simulink model "s32k344_mcb_open_loop_s32ct"  (R2024b)
settings: Solver=FixedStepAuto  StartTime=0.0  StopTime=10.0  RelTol=1e-3  EnableMultiTasking=on
PreLoadFcn:
  | % NXP_MBDT_S32K3 callback: DO NOT REMOVE
  | mbd_s32k3.common.nxp.model_callbacks.preLoadFcn();
  | 
  | s32k344Data;
  | mcbOpenLoopData;
PostLoadFcn:
  | % NXP_MBDT_S32K3 callback: DO NOT REMOVE
  | mbd_s32k3.common.nxp.model_callbacks.postLoadFcn();
InitFcn:
  | % NXP_MBDT_S32K3 callback: DO NOT REMOVE
  | mbd_s32k3.common.nxp.model_callbacks.initFcn();
values from neighbouring files (symbols this model uses):
  PWM_DutyScale = 32768    [s32k344Data.m]
  PWM_Period = 8000    [s32k344Data.m]
  Ts_motor = T_pwm    (= 5e-05)    [s32k344Data.m]
undefined symbols (not defined in the file or in its folder): inverter, LogicOutputId, pmsm, Value
libraries: mbd_s32k3_io_library x14, mbd_s32k3_cdd_library x4, simulink x4, mbd_s32k3_isr_library x1, mbd_s32k3_utility_library x1
(part 1 of 3)
Description:
  | Motor Control PMSM Open Loop MCB S32CT
  | 
  | 
  |             <script src="../../../../doc/src/utils.js">
  | 
  |             <script src="../../../../doc/src/details_summary_utils.js">
  | 
  |             <script src="../../../../doc/src/matlab_command_link.js">
  | 
  |             <link rel="stylesheet" type="text/css" href="../../../../doc/style.css">
  | 
  | 
  | 
  | 
  |         Motor Control PMSM Open Loop MCB S32CT
  |         <a class="matlab-command" href="matlab:open('s32k344_mcb_open_loop_s32ct')"><button class="matlab-command" style=" --data-title: ' Run MATLAB command: open(\'s32k344_mcb_open_loop_s32ct')'">Open Example
  |         The s32k344_mcb_open_loop_s32ct.mdl example illustrates how the MCSPTE1AK344 Motor Control Development Kit is used to run a motor by achieving an open-loop control algorithm (also known as scalar control or V/Hz control). This technique varies the stator voltage and frequency to control the rotor speed without using any feedback from the motor. Open-Loop control does not have the ability to consider the external conditions that can affect the motor speed. Therefore, the control system cannot automatically correct the deviation between the desired and the actual motor speed. This Simulink® model is configured to work with both Sunrise 42BLY3A78-24110 and Linix 45ZWN24-40 motors and it has been tested on the S32K3X4EVB-Q172 RevA board.
  | 
  |             This model shows how to get started with Motor Control Blockset™ and verify the hardware setup for the MCSPTE1AK344 Development Kit by running the motor. The model algorithm also reads the ADC values for the 3-phase currents and DC Bus voltage, using the hardware triggering scheme of eMIOS-TRGMUX-BCTU-ADC. To generate the output commands for spinning the motor, this model uses the Motor Control Blockset™ Library. The FreeMASTER application is used to connect to the running on-target algorithm using the FreMASTER CMSIS-DAP Communication Plug-in.
  | 
  |             Note: If there is no error, the <b style="color:blue">RGBLED0_BLUE will be on which means the application is waiting for the user commands. If there is any error, the motor will not run, and the <b style="color:red">RGBLED0_RED will stay on. If the motor is spinning and no fault is detected, the <b style="color:green">RGBLED0_GREEN will stay on.
  | 
  |             Note: Make sure to have included in MATLAB Path the mcat_src_files directory!
  | 
  |         Toolchain Supported
  | 
  | 
  |                 S32 Design Studio 3.5
  | 
  | 
  |         Required Hardware
  | 
  | 
  |                 Personal Computer
  | 
  |                 <a href="https://www.nxp.com/design/development-boards/automotive-motor-control-solutions/arm-based-solutions-/s32k344-brushless-direct-current-and-permanent-magnet-synchronous-motor-control-development-kit:MCSPTE1AK344"> MCSPTE1AK344 BLDC and PMSM Motor Control Development Kit<img src="../img/MCSPTE1AK344.jpg" alt="Motor Control PMSM Open Loop MCB S32CT" height="auto"> The MCSPTE1AK344 Development kit contains:  <a href="https://www.nxp.com/design/development-boards/automotive-development-platforms/hardware-tools-accessories/motor-control-shield-for-devkit:DEVKIT-MOTORGD"> DEVKIT-MOTORGD board<a href="https://www.nxp.com/design/design-center/development-boards/automotive-development-platforms/s32k-mcu-platforms/s32k3x4evb-t172-evaluation-board-for-automotive-general-purpose:S32K3X4EVB-T172">S32K3X4EVB-T172 board or <a href="https://www.nxp.com/design/development-boards/automotive-development-platforms/s32k-mcu-platforms/s32k3x4-q172-general-purpose-development-board:S32K3X4EVB-Q172">S32K3X4EVB-Q172 board<a href="https://www.sunrisemotor-cn.com/Product/142451.html"> Sunrise 42BLY3A78-24110 Motor
  | 
  |                 12V Power Supply
  | 
  |                 Micro USB cable
  | 
  | 
  |         Prepare the Demo
  | 
  | 
  |                 The MCSPTE1AK344 kit has different resistors removed/populated compared with the original S32K3X4EVB board. The following table presents all the modifications needed for the S32K3X4EVB boards to work with all MBDT BLDC/PMSM models:<table class="tg" style="undefined;table-layout: fixed; width: 700px"><col style="width: 182.px"><col style="width: 144.px"><col style="width: 112.px"><col style="width: 144.px"><col style="width: 112.px">Board RevisionsRemoved resistorsValue/PackagePopulated resistorsValue/Package<td rowspan="2">S32K3X4EVB-T172R37, R4010k Ohm/0402<td rowspan="2">R255, R257, R2273<td rowspan="2">0 Ohm/0402R22390 Ohm/0402<td rowspan="2">S32K3X4EVB-Q172 RevAR37, R4010k Ohm/0402<td rowspan="2">R255, R257<td rowspan="2">0 Ohm/0402R91, R960 Ohm/0402<td rowspan="2">S32K3X4EVB-Q172 RevBR37, R4010k Ohm/0402<td rowspan="2">R255, R257, R2188<td rowspan="2">0 Ohm/0402R91, R96, R21860 Ohm/0402
  | 
  |                 For more details check the <a href="https://www.nxp.com/webapp/Download?colCode=S32K3X4EVBBMUG&location=null">S32K3X4EVB-Q172 Board Modifications for MCSPTE1AK344 Motor Control Kit Schematic Addendum.
  | 
  |                 To get started on the MCSPTE1AK344 kit visit the website <a href="https://www.nxp.com/document/guide/get-started-with-the-mcspte1ak344-development-kit:GS-MCSPTE1AK344"> Get Started with the MCSPTE1AK344 Development Kit.
  | 
  |                 The connections between the S32K3X4EVB board and the DEVKIT-MOTORGD can be found in the following table:<img src="../img/Headers_pinout.jpg" alt="Motor Control PMSM Open Loop MCB S32CT" height="500px" >
  | 
  |                 Overview of the location of USER_SW0/SW1, RGBLED0, 12 Vin DC power, USB J40 connector, SW1 for powering ON, board jumpers J8, J9, J10, and J11:<img src="../img/MCSPTE1AK344_top.jpg" alt="Motor Control PMSM Open Loop MCB S32CT" height="500px" >
  | 
  |                 Take a closer look and check the DEVKIT-MOTORGD jumpers J9, J10, and J11 are in positions 2-1 and J8 is open, this configuration works with all MBDT BLDC/PMSM models:<img src="../img/PINS_J9_J11.jpg" alt="Motor Control PMSM Open Loop MCB S32CT" height="300px" >
  | 
  |                 Connect a micro-USB cable between the host PC and the OpenSDA USB port (J40) and switch the SW1 to position 2 on the S32K3X4EVB board.
  | 
  |                 Connect the 12V Power supply to the DEVKIT-MOTORGD board and switch the SW1 from the 2 position to the 1 position on the S32K3X4EVB board: <img src="../img/Plug-Power.jpg" alt="Motor Control PMSM Open Loop MCB S32CT" height="300px">
  | 
  |                 The four LEDs next to SW1 will power on and be solid orange, if they are blinking, move the switch from position 1 to 2 and back to position 1 to start the SBC without the active watchdog.
  | 
  |                 Open the s32k344_mcb_open_loop_s32ct.mdl model.Users can choose between the Sunrise 42BLY3A78-24110 or the Linix 45ZWN24-40 motor from <a href="https://www.nxp.com/design/design-center/development-boards-and-designs/general-purpose-mcus/low-voltage-3-phase-motor-for-frdm-platform:FRDM-MC-LVMTR"> the NXP page.
  | 
  |                 Click on "Generate Code, Build & Deploy" to download the program to the target board and the <b style="color:blue">RGBLED0_BLUE lights up.
  | 
  |                 To open the FreeMASTER software click on "4. Open the FreeMASTER project" from inside the Simulink model, this will open the "s32k344_mcb_open_loop_s32ct.pmpx" file in the "FreeMASTER_control" folder.
  | 
  |                 Click on the "GO" buton (or press CTRL+G) to enable FreeMASTER communication with the S32K3X4EVB board:<img src="../img/FM_Start.jpg" alt="Motor Control PMSM Open Loop MCB S32CT" height="150px"> Successful communication displays in the status bar at the bottom as: RS232; port = COMn; speed = 115200.
  | 
  | 
  |         Running the Demo
  | 
  | 
  |                 To validate this example, please follow the steps below:   To start the motor, set the Enable variable from 0 to 1. The Desired speed can be set from FreeMASTER project with values between -1000 and 1000 RPM The DC Bus voltage, 3-phase currents and generated PWM signals could be also checked in FreeMASTER; The <b style="color:green">RGBLED0_GREEN will be ON when the motor spins:<img src="../img/PMSM.gif" alt="Motor Control PMSM Open Loop MCB S32CT" height="100">
  | 
  | 
  |         Customization Options
  | 
  | 
  |                 For changing the processor, the configuration tool, and for creating custom configuration projects, please visit section 3.6 of Release Notes <a class="pdf-link" href="../../../../doc/docs/manual/Model_Based_Design_Toolbox_S32K3_Series_Release_Notes.pdf">Model_Based_Design_Toolbox_S32K3_Series_Release_Notes.pdf
  | 
  |                 For S32K3 Design Tools and Files, please visit <a href="https://www.nxp.com/products/processors-and-microcontrollers/arm-microcontrollers/s32k-automotive-mcus/s32k3-microcontrollers-for-general-purpose:S32K3">S32K3 Microcontrollers
settings Model: DataDictionary=s32k344_mcb_open_loop_s32ct.sldd  Creator=nxf35401  LastModifiedBy=nxf64875
settings SolverCC: AlgebraicLoopSolver=TrustRegion
settings DataIOCC: LimitDataPoints=on  SaveFormat=Array  SaveOutput=off  SaveTime=off  ReturnWorkspaceOutputs=off
settings OptimizationCC: DefaultParameterBehavior=Inlined  UseFloatMulNetSlope=on  DefaultUnderspecifiedDataType=single  EnhancedBackFolding=on  PassReuseOutputArgsAs=Individual arguments  ZeroExternalMemoryAtStartup=off  ZeroInternalMemoryAtStartup=off  NoFixptDivByZeroProtection=on  EfficientFloat2IntCast=on  MaxStackSize=128  SimCompilerOptimization=on  EfficientTunableParamExpr=on
settings DebuggingCC: InheritedTsInSrcMsg=none  MultiTaskDSMMsg=none  MultiTaskRateTransMsg=warning  ParameterPrecisionLossMsg=none  ParameterTunabilityLossMsg=error  UnconnectedInputMsg=warning  UnconnectedOutputMsg=warning  UnconnectedLineMsg=warning
settings HardwareCC: ProdBitPerPointer=32  ProdBitPerSizeT=32  ProdBitPerPtrDiffT=32  ProdLargestAtomicInteger=Long  ProdLargestAtomicFloat=Double  ProdWordSize=32  ProdHWDeviceType=ARM Compatible->ARM Cortex
settings ModelReferenceCC: EnableRefExpFcnMdlSchedulingChecks=on
settings SFSimCC: MATLABDynamicMemAlloc=off
settings RTWCC: Description=Embedded Coder  SystemTargetFile=ert.tlc  HardwareBoard=NXP S32K3xx  TemplateMakefile=ert_default_tmf  Toolchain=S32DS GCC  BuildConfiguration=Faster Runs  IncludeHyperlinkInReport=on  GPUComputeCapability=3.5  DLArmComputeVersion=19.05
settings CodeAppCC: ForceParamTrailComments=on  IgnoreCustomStorageClasses=off  OperatorAnnotations=on  SimulinkDataObjDesc=on  SFDataObjDesc=on  InsertBlockDesc=on  StateflowObjectComments=on
settings ERTTargetCC: TargetLangStandard=C99 (ISO)  SupportNonFinite=off  SupportComplex=off  InlinedParameterPlacement=Hierarchical  ERTSrcFileBannerTemplate=mbd_s32k3_ert_code_template.cgt  ERTHdrFileBannerTemplate=mbd_s32k3_ert_code_template.cgt  ERTDataSrcFileTemplate=mbd_s32k3_ert_code_template.cgt  ERTDataHdrFileTemplate=mbd_s32k3_ert_code_template.cgt  DynamicArrayContainerType=coder::array

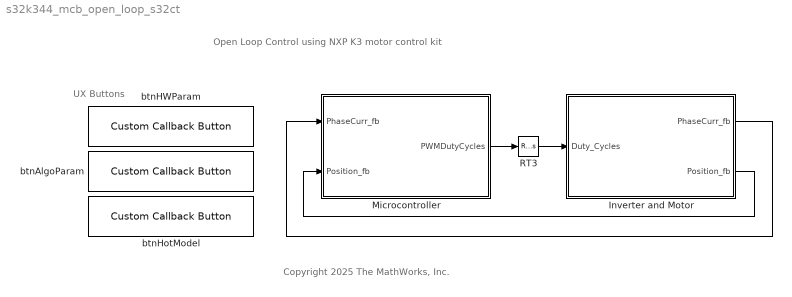
== system s32k344_mcb_open_loop_s32ct ==
  note: UX Buttons
  note: Open Loop Control using NXP K3 motor control kit
  note: Copyright 2025 The MathWorks, Inc.
  Inverter and Motor : Subsystem
  Microcontroller : Subsystem
  RT3 : RateTransition  Integrity=off
  btnAlgoParam : CustomCallbackButton  Configuration="{\"components\":[{\"name\":\"BackgroundImageComponent\",\"settings\":{\"image\":{\"size\":[0,0],\"src\":\"default\",\"srcOrientation\":\"Right\"},\"position\":[0,0,1,1]}},{\"name\":\"ButtonStateComponent\",\"settings\":{\"buttonType\":\"momentary\",\"clickFcn\":\"edit mcbOpenLoopData.m;\",\"onValue\":1,\"position\":[0,0,1,1],\"pressDelay\":\"500\",\"pressFcn\":\"\",\"repeatInterval\":\"0\",\"states\":[{\"horizontalAlignment\":\"center\",\"image\":{\"position\":[0,0,1,1],\"size\":[1,1],\"src\":\"default\",\"srcOrientation\":\"Right\"},\"label\":{\"color\":[0.01176470588,0.01176470588,0.01176470588,1],\"icon\":{\"size\":[0,0],\"src\":\"default\",\"srcOrientation\":\"Right\"},\"iconOffset\":0,\"iconPlacement\":\"left\",\"opacity\":1,\"show\":true,\"text\":{\"content\":\"Edit motor and algorithm parameters\",\"font\":\"Helvetica\"}},\"labelOffset\":[0,0],\"verticalAlignment\":\"middle\"},{\"horizontalAlignment\":\"center\",\"image\":{\"position\":[0,0,1,1],\"size\":[1,1],\"src\":\"default\",\"srcOrientation\":\"Right\"},\"label\":{\"color\":[0.01176470588,0.01176470588,0.01176470588,1],\"icon\":{\"size\":[0,0],\"src\":\"default\",\"srcOrientation\":\"Right\"},\"iconOffset\":0,\"iconPlacement\":\"left\",\"opacity\":1,\"show\":true,\"text\":{\"content\":\"Edit motor and algorithm parameters\",\"font\":\"Helvetica\"}},\"labelOffset\":[0,0],\"verticalAlignment\":\"middle\"},{\"horizontalAlignment\":\"center\",\"image\":{\"position\":[0,0,1,1],\"size\":[1,1],\"src\":\"default\",\"srcOrientation\":\"Right\"},\"label\":{\"color\":[0.01176470588,0.01176470588,0.01176470588,1],\"icon\":{\"size\":[0,0],\"src\":\"default\",\"srcOrientation\":\"Right\"},\"iconOffset\":0,\"iconPlacement\":\"left\",\"opacity\":1,\"show\":true,\"text\":{\"content\":\"Edit motor and algorithm parameters\",\"font\":\"Helvetica\"}},\"labelOffset\":[0,0],\"verticalAlignment\":\"middle\"},{\"horizontalAlignment\":\"center\",\"image\":{\"position\":[0,0,1,1],\"size\":[1,1],\"src\":\"default\",\"srcOrientation\":\"Right\"},\"label\":{\"color\":[0.01176470588,0.01176470588,0.01176470588,1],\"icon\":{\"size\":[0,0],\"src\":\"default\",\"srcOrientation\":\"Right\"},\"iconOffset\":0,\"iconPlacement\":\"left\",\"opacity\":1,\"show\":true,\"text\":{\"content\":\"Edit motor and algorithm parameters\",\"font\":\"Helvetica\"}},\"labelOffset\":[0,0],\"verticalAlignment\":\"middle\"}]}},{\"name\":\"ForegroundImageComponent\",\"settings\":{\"image\":{\"size\":[0,0],\"src\":\"default\",\"srcOrientation\":\"Right\"},\"isForeground\":1,\"position\":[0,0,1,1]}}],\"settings\":{\"BindingType\":\"standalone\",\"backgroundColor\":[244,244,244,1],\"backgroundOffset\":0.2,\"backgroundOpacity\":1,\"fixedAspectRatio\":\"off\",\"foregroundColor\":[0.01176470588,0.01176470588,0.01176470588,1],\"migratedFromLegacy\":true,\"useBackgroundColor\":true,\"variant\":\"callback\",\"version\":\"R2024b\"},\"type\":\"Button\"}"  CustomBackgroundColor="{\"color\":[0.9568627451,0.9568627451,0.9568627451],\"show\":true}"
  btnHWParam : CustomCallbackButton  Configuration="{\"components\":[{\"name\":\"BackgroundImageComponent\",\"settings\":{\"image\":{\"size\":[0,0],\"src\":\"default\",\"srcOrientation\":\"Right\"},\"position\":[0,0,1,1]}},{\"name\":\"ButtonStateComponent\",\"settings\":{\"buttonType\":\"momentary\",\"clickFcn\":\"edit s32k344Data.m;\",\"onValue\":1,\"position\":[0,0,1,1],\"pressDelay\":\"500\",\"pressFcn\":\"\",\"repeatInterval\":\"0\",\"states\":[{\"horizontalAlignment\":\"center\",\"image\":{\"position\":[0,0,1,1],\"size\":[1,1],\"src\":\"default\",\"srcOrientation\":\"Right\"},\"label\":{\"color\":[0.01176470588,0.01176470588,0.01176470588,1],\"icon\":{\"size\":[0,0],\"src\":\"default\",\"srcOrientation\":\"Right\"},\"iconOffset\":0,\"iconPlacement\":\"left\",\"opacity\":1,\"show\":true,\"text\":{\"content\":\"Edit hardware parameters\",\"font\":\"Helvetica\"}},\"labelOffset\":[0,0],\"verticalAlignment\":\"middle\"},{\"horizontalAlignment\":\"center\",\"image\":{\"position\":[0,0,1,1],\"size\":[1,1],\"src\":\"default\",\"srcOrientation\":\"Right\"},\"label\":{\"color\":[0.01176470588,0.01176470588,0.01176470588,1],\"icon\":{\"size\":[0,0],\"src\":\"default\",\"srcOrientation\":\"Right\"},\"iconOffset\":0,\"iconPlacement\":\"left\",\"opacity\":1,\"show\":true,\"text\":{\"content\":\"Edit hardware parameters\",\"font\":\"Helvetica\"}},\"labelOffset\":[0,0],\"verticalAlignment\":\"middle\"},{\"horizontalAlignment\":\"center\",\"image\":{\"position\":[0,0,1,1],\"size\":[1,1],\"src\":\"default\",\"srcOrientation\":\"Right\"},\"label\":{\"color\":[0.01176470588,0.01176470588,0.01176470588,1],\"icon\":{\"size\":[0,0],\"src\":\"default\",\"srcOrientation\":\"Right\"},\"iconOffset\":0,\"iconPlacement\":\"left\",\"opacity\":1,\"show\":true,\"text\":{\"content\":\"Edit hardware parameters\",\"font\":\"Helvetica\"}},\"labelOffset\":[0,0],\"verticalAlignment\":\"middle\"},{\"horizontalAlignment\":\"center\",\"image\":{\"position\":[0,0,1,1],\"size\":[1,1],\"src\":\"default\",\"srcOrientation\":\"Right\"},\"label\":{\"color\":[0.01176470588,0.01176470588,0.01176470588,1],\"icon\":{\"size\":[0,0],\"src\":\"default\",\"srcOrientation\":\"Right\"},\"iconOffset\":0,\"iconPlacement\":\"left\",\"opacity\":1,\"show\":true,\"text\":{\"content\":\"Edit hardware parameters\",\"font\":\"Helvetica\"}},\"labelOffset\":[0,0],\"verticalAlignment\":\"middle\"}]}},{\"name\":\"ForegroundImageComponent\",\"settings\":{\"image\":{\"size\":[0,0],\"src\":\"default\",\"srcOrientation\":\"Right\"},\"isForeground\":1,\"position\":[0,0,1,1]}}],\"settings\":{\"BindingType\":\"standalone\",\"backgroundColor\":[244,244,244,1],\"backgroundOffset\":0.2,\"backgroundOpacity\":1,\"fixedAspectRatio\":\"off\",\"foregroundColor\":[0.01176470588,0.01176470588,0.01176470588,1],\"migratedFromLegacy\":true,\"useBackgroundColor\":true,\"variant\":\"callback\",\"version\":\"R2024b\"},\"type\":\"Button\"}"  CustomBackgroundColor="{\"color\":[0.9568627451,0.9568627451,0.9568627451],\"show\":true}"
  btnHotModel : CustomCallbackButton  Configuration="{\"components\":[{\"name\":\"BackgroundImageComponent\",\"settings\":{\"image\":{\"size\":[0,0],\"src\":\"default\",\"srcOrientation\":\"Right\"},\"position\":[0,0,1,1]}},{\"name\":\"ButtonStateComponent\",\"settings\":{\"buttonType\":\"momentary\",\"clickFcn\":\"OpenLoopControlHost;\",\"onValue\":1,\"position\":[0,0,1,1],\"pressDelay\":\"500\",\"pressFcn\":\"\",\"repeatInterval\":\"0\",\"states\":[{\"horizontalAlignment\":\"center\",\"image\":{\"position\":[0,0,1,1],\"size\":[1,1],\"src\":\"default\",\"srcOrientation\":\"Right\"},\"label\":{\"color\":[0.01176470588,0.01176470588,0.01176470588,1],\"icon\":{\"size\":[0,0],\"src\":\"default\",\"srcOrientation\":\"Right\"},\"iconOffset\":0,\"iconPlacement\":\"left\",\"opacity\":1,\"show\":true,\"text\":{\"content\":\"Open host model\",\"font\":\"Helvetica\"}},\"labelOffset\":[0,0],\"verticalAlignment\":\"middle\"},{\"horizontalAlignment\":\"center\",\"image\":{\"position\":[0,0,1,1],\"size\":[1,1],\"src\":\"default\",\"srcOrientation\":\"Right\"},\"label\":{\"color\":[0.01176470588,0.01176470588,0.01176470588,1],\"icon\":{\"size\":[0,0],\"src\":\"default\",\"srcOrientation\":\"Right\"},\"iconOffset\":0,\"iconPlacement\":\"left\",\"opacity\":1,\"show\":true,\"text\":{\"content\":\"Open host model\",\"font\":\"Helvetica\"}},\"labelOffset\":[0,0],\"verticalAlignment\":\"middle\"},{\"horizontalAlignment\":\"center\",\"image\":{\"position\":[0,0,1,1],\"size\":[1,1],\"src\":\"default\",\"srcOrientation\":\"Right\"},\"label\":{\"color\":[0.01176470588,0.01176470588,0.01176470588,1],\"icon\":{\"size\":[0,0],\"src\":\"default\",\"srcOrientation\":\"Right\"},\"iconOffset\":0,\"iconPlacement\":\"left\",\"opacity\":1,\"show\":true,\"text\":{\"content\":\"Open host model\",\"font\":\"Helvetica\"}},\"labelOffset\":[0,0],\"verticalAlignment\":\"middle\"},{\"horizontalAlignment\":\"center\",\"image\":{\"position\":[0,0,1,1],\"size\":[1,1],\"src\":\"default\",\"srcOrientation\":\"Right\"},\"label\":{\"color\":[0.01176470588,0.01176470588,0.01176470588,1],\"icon\":{\"size\":[0,0],\"src\":\"default\",\"srcOrientation\":\"Right\"},\"iconOffset\":0,\"iconPlacement\":\"left\",\"opacity\":1,\"show\":true,\"text\":{\"content\":\"Open host model\",\"font\":\"Helvetica\"}},\"labelOffset\":[0,0],\"verticalAlignment\":\"middle\"}]}},{\"name\":\"ForegroundImageComponent\",\"settings\":{\"image\":{\"size\":[0,0],\"src\":\"default\",\"srcOrientation\":\"Right\"},\"isForeground\":1,\"position\":[0,0,1,1]}}],\"settings\":{\"BindingType\":\"standalone\",\"backgroundColor\":[244,244,244,1],\"backgroundOffset\":0.2,\"backgroundOpacity\":1,\"fixedAspectRatio\":\"off\",\"foregroundColor\":[0.01176470588,0.01176470588,0.01176470588,1],\"migratedFromLegacy\":true,\"useBackgroundColor\":true,\"variant\":\"callback\",\"version\":\"R2024b\"},\"type\":\"Button\"}"  CustomBackgroundColor="{\"color\":[0.9568627451,0.9568627451,0.9568627451],\"show\":true}"
  wires:
  Inverter and Motor/1(PhaseCurr_fb) -> Microcontroller/1(PhaseCurr_fb)
  RT3/1 -> Inverter and Motor/1(Duty_Cycles)
  Microcontroller/1(PWMDutyCycles) -> RT3/1
  Inverter and Motor/2(Position_fb) -> Microcontroller/2(Position_fb)

== system s32k344_mcb_open_loop_s32ct/Inverter and Motor ==
  Duty_Cycles : Inport
  Inverter and Motor : Subsystem  Variant=on  VariantControlMode=sim codegen switching
  PhaseCurr_fb : Outport
  Position_fb : Outport  Port=2
  wires:
  Inverter and Motor/1(PhaseCurr_fb) -> PhaseCurr_fb/1
  Inverter and Motor/2(Position_fb) -> Position_fb/1
  Duty_Cycles/1 -> Inverter and Motor/1(Duty_Cycles)

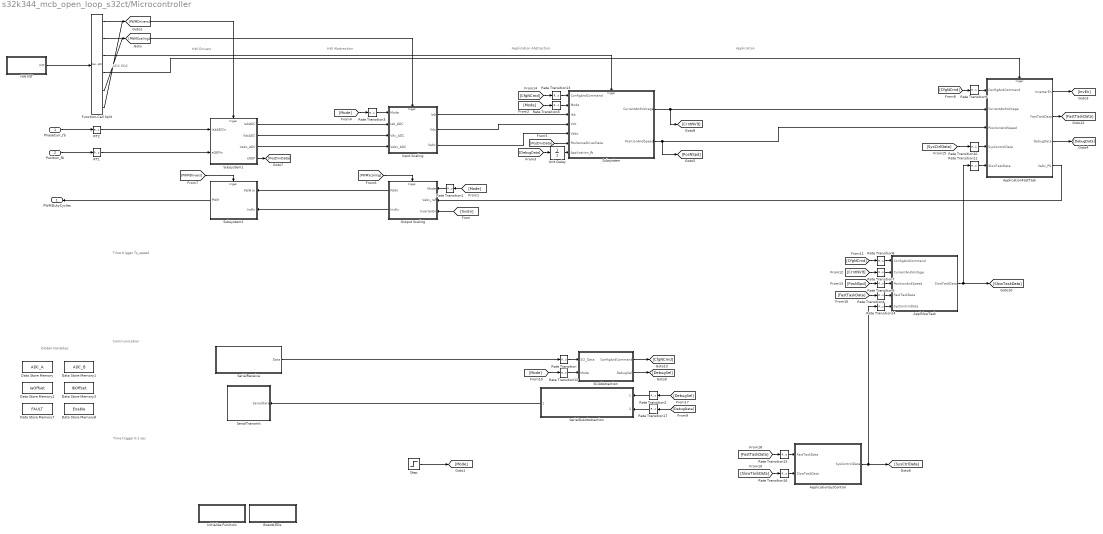
== system s32k344_mcb_open_loop_s32ct/Microcontroller ==
  note: Time trigger Ts_speed
  note: HW Abstraction
  note: Time trigger 0.1 sec
  note: Application
  note: HW Drivers
  note: Communication
  note: ADC EOC
  note: Application Abstraction
  note: Global Variables:
  PhaseCurr_fb : Inport
  Position_fb : Inport  Port=2
  ApplSlowTask : Subsystem
  ApplicationFastTask : Subsystem
  ApplicationSysControl : Subsystem
  BoardLEDs : Subsystem
  Data Store Memory : DataStoreMemory  DataStoreName=ADC_A  ShowAdditionalParam=off  OutDataTypeStr=single
  Data Store Memory1 : DataStoreMemory  DataStoreName=ADC_B  ShowAdditionalParam=off  OutDataTypeStr=single
  Data Store Memory2 : DataStoreMemory  DataStoreName=IaOffset  InitialValue=inverter.AOffset  ShowAdditionalParam=off
  Data Store Memory3 : DataStoreMemory  DataStoreName=IbOffset  InitialValue=inverter.BOffset  ShowAdditionalParam=off
  Data Store Memory7 : DataStoreMemory  DataStoreName=FAULT  WriteAfterWriteMsg=warning  WriteAfterReadMsg=warning  ShowAdditionalParam=off  OutDataTypeStr=boolean
  Data Store Memory8 : DataStoreMemory  DataStoreName=Enable  ReadBeforeWriteMsg=warning  WriteAfterWriteMsg=warning  WriteAfterReadMsg=warning  ShowAdditionalParam=off  OutDataTypeStr=boolean
  Function-Call Split : FunctionCallSplit  IconShape=distinctive  NumOutputPorts=6
  HW INT : Subsystem  Variant=on  VariantControlMode=sim codegen switching
  Initialize Function : Subsystem  TreatAsAtomicUnit=on
  Input Scaling : Subsystem
  Output Scaling : Subsystem
  RT1 : RateTransition  Deterministic=off
  RT2 : RateTransition  Deterministic=off
  Rate Transition : RateTransition  Deterministic=off
  Rate Transition{1,3,5,9..11,13} (7 alike) : RateTransition  Deterministic=off  OutPortSampleTime=Ts
  Rate Transition12 : RateTransition  Deterministic=off
  Rate Transition{4,6..8,14} (5 alike) : RateTransition  Deterministic=off  OutPortSampleTime=Ts_speed
  Rate Transition15 : RateTransition  Deterministic=off  OutPortSampleTime=0.1
  Rate Transition16 : RateTransition  Deterministic=off  OutPortSampleTime=0.1
  Rate Transition17 : RateTransition  Deterministic=off  OutPortSampleTime=0.01
  Rate Transition2 : RateTransition  Deterministic=off  OutPortSampleTime=0.01
  SCIAbstraction : Subsystem
  SerialOutAbstraction : Subsystem  ReferencedSubsystem=SCIOutAbstractionOpenLoop
  SerialReceive : Subsystem  TreatAsAtomicUnit=on  SystemSampleTime=0.1
  SerialTransmit : Subsystem  TreatAsAtomicUnit=on  SystemSampleTime=0.01
  Step : Step  After=2  OutDataTypeStr=single  SampleTime=0.1
  Subsystem : Subsystem
  Subsystem1 : Subsystem
  Subsystem2 : Subsystem
  Unit Delay : UnitDelay  SampleTime=-1  HasFrameUpgradeWarning=on
  PWMDutyCycles : Outport
  wires:
  ApplicationFastTask/1(InverterEn) -> [InvEn]
  [InvEn] -> Output Scaling/3(InverterEn)
  ApplicationFastTask/4(Vabc_PU) -> Output Scaling/2(Vabc_ref)
  Step/1 -> [Mode]
  [Mode] -> Rate Transition1/1
  [Mode] -> Rate Transition5/1
  ApplicationFastTask/3(DebugData) -> [DebugData]
  [DebugData] -> Unit Delay/1
  Subsystem/1(CurrentAndVoltage) -> [CrntNVlt], ApplicationFastTask/2(CurrentAndVoltage)
  Rate Transition5/1 -> Subsystem/2(Mode)
  Input Scaling/1(Iab) -> Subsystem/3(Iab)
  Input Scaling/2(Vdc) -> Subsystem/4(Vdc)
  Input Scaling/3(Vabc) -> Subsystem/5(Vabc)
  Unit Delay/1 -> Subsystem/7(Application_fb)
  Subsystem/2(PositionAndSpeed) -> [PosNSpd], ApplicationFastTask/3(PositionAndSpeed)
  Rate Transition3/1 -> Input Scaling/1(Mode)
  [Mode] -> Rate Transition3/1
  [PosDrvData] -> Subsystem/6(PosSenseDriverData)
  PhaseCurr_fb/1 -> RT2/1
  Position_fb/1 -> RT1/1
  Subsystem1/1(IabADC) -> Input Scaling/2(Iab_ADC)
  Subsystem1/2(VdcADC) -> Input Scaling/3(Vdc_ADC)
  Subsystem1/3(Vabc_ADC) -> Input Scaling/4(Vabc_ADC)
  Subsystem1/4(eQEP) -> [PosDrvData]
  Output Scaling/1(PWM) -> Subsystem2/1(PWM In)
  Output Scaling/2(InvEn) -> Subsystem2/2(InvEn)
  Subsystem2/1(PWM) -> PWMDutyCycles/1
  Function-Call Split/1 -> Subsystem1/Trigger
  Function-Call Split/3 -> Subsystem/Trigger
  Function-Call Split/2 -> Input Scaling/Trigger
  Function-Call Split/4 -> ApplicationFastTask/Trigger
  Function-Call Split/5 -> [PWMScaling]
  [PWMScaling] -> Output Scaling/Trigger
  Function-Call Split/6 -> [PWMDrivers]
  [PWMDrivers] -> Subsystem2/Trigger
  Rate Transition11/1 -> ApplicationFastTask/5(SlowTaskData)
  ApplSlowTask/1(SlowTaskData) -> Rate Transition11/1, [SlowTaskData]
  [FastTaskData] -> Rate Transition15/1
  [SlowTaskData] -> Rate Transition16/1
  Rate Transition15/1 -> ApplicationSysControl/1(FastTaskData)
  Rate Transition16/1 -> ApplicationSysControl/2(SlowTaskData)
  Rate Transition14/1 -> ApplSlowTask/5(SysControlData)
  ApplicationSysControl/1(SysControlData) -> [SysCtrlData], Rate Transition14/1
  Rate Transition4/1 -> ApplSlowTask/4(FastTaskData)
  Rate Transition6/1 -> ApplSlowTask/3(PositionAndSpeed)
  Rate Transition7/1 -> ApplSlowTask/2(CurrentAndVoltage)
  Rate Transition8/1 -> ApplSlowTask/1(ConfigAndCommand)
  [CfgNCmd] -> Rate Transition8/1
  [CrntNVlt] -> Rate Transition7/1
  [PosNSpd] -> Rate Transition6/1
  [FastTaskData] -> Rate Transition4/1
  [CfgNCmd] -> Rate Transition9/1
  Rate Transition9/1 -> ApplicationFastTask/1(ConfigAndCommand)
  [SysCtrlData] -> Rate Transition10/1
  Rate Transition10/1 -> ApplicationFastTask/4(SysControlData)
  ApplicationFastTask/2(FastTaskData) -> [FastTaskData]
  SCIAbstraction/1(ConfigAndCommand) -> [CfgNCmd]
  SCIAbstraction/2(DebugSel) -> [DebugSel]
  Rate Transition/1 -> SCIAbstraction/1(SCI_Data)
  Rate Transition12/1 -> SCIAbstraction/2(Mode)
  [Mode] -> Rate Transition12/1
  SerialReceive/1(Data) -> Rate Transition/1
  Rate Transition13/1 -> Subsystem/1(ConfigAndCommand)
  [CfgNCmd] -> Rate Transition13/1
  RT2/1 -> Subsystem1/1(IabADCIn)
  RT1/1 -> Subsystem1/2(eQEPIn)
  Rate Transition1/1 -> Output Scaling/1(Mode)
  HW INT/1(INT) -> Function-Call Split/1
  SerialOutAbstraction/1 -> SerialTransmit/1(SerialData)
  Rate Transition2/1 -> SerialOutAbstraction/1
  Rate Transition17/1 -> SerialOutAbstraction/2
  [DebugData] -> Rate Transition17/1
  [DebugSel] -> Rate Transition2/1

== system s32k344_mcb_open_loop_s32ct/Inverter and Motor/Inverter and Motor ==
  Duty_Cycles : Inport
  Codegen : Subsystem  VariantControl=(codegen)
  Sim : Subsystem  VariantControl=(sim)
  PhaseCurr_fb : Outport
  Position_fb : Outport  Port=2

== system s32k344_mcb_open_loop_s32ct/Microcontroller/ApplSlowTask ==
  ConfigAndCommand : Inport
  CurrentAndVoltage : Inport  Port=2
  PositionAndSpeed : Inport  Port=3
  FastTaskData : Inport  Port=4
  SysControlData : Inport  Port=5
  SlowTask : Subsystem  ReferencedSubsystem=ApplicationOpenLoopLowPrio
  SlowTaskData : Outport
  wires:
  SlowTask/1 -> SlowTaskData/1
  FastTaskData/1 -> SlowTask/4
  CurrentAndVoltage/1 -> SlowTask/2
  ConfigAndCommand/1 -> SlowTask/1
  PositionAndSpeed/1 -> SlowTask/3
  SysControlData/1 -> SlowTask/5

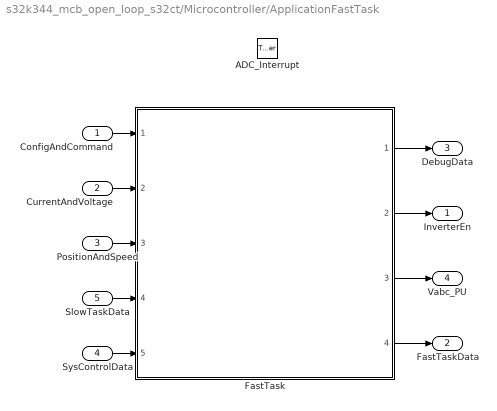
== system s32k344_mcb_open_loop_s32ct/Microcontroller/ApplicationFastTask ==
  ConfigAndCommand : Inport
  CurrentAndVoltage : Inport  Port=2
  PositionAndSpeed : Inport  Port=3
  SysControlData : Inport  Port=4
  SlowTaskData : Inport  Port=5
  ADC_Interrupt : TriggerPort  TriggerType=function-call  VariantControl=(inherit)
  FastTask : Subsystem  ReferencedSubsystem=ApplicationOpenLoopHighPrio
  InverterEn : Outport
  FastTaskData : Outport  Port=2
  DebugData : Outport  Port=3
  Vabc_PU : Outport  Port=4
  wires:
  SysControlData/1 -> FastTask/5
  FastTask/3 -> Vabc_PU/1
  SlowTaskData/1 -> FastTask/4
  FastTask/2 -> InverterEn/1
  FastTask/4 -> FastTaskData/1
  ConfigAndCommand/1 -> FastTask/1
  CurrentAndVoltage/1 -> FastTask/2
  PositionAndSpeed/1 -> FastTask/3
  FastTask/1 -> DebugData/1

== system s32k344_mcb_open_loop_s32ct/Microcontroller/ApplicationSysControl ==
  FastTaskData : Inport
  SlowTaskData : Inport  Port=2
  SysControl : Subsystem  TreatAsAtomicUnit=on  SystemSampleTime=0.1  ReferencedSubsystem=ApplicationOpenLoopSysControl
  SysControlData : Outport
  wires:
  SlowTaskData/1 -> SysControl/2
  SysControl/1 -> SysControlData/1
  FastTaskData/1 -> SysControl/1

== system s32k344_mcb_open_loop_s32ct/Microcontroller/BoardLEDs ==
  Data Store Read1 : DataStoreRead  DataStoreName=FAULT  IndexOptions=Index vector (dialog)  Indices=1  OutputSizes=1
  Fault_LED : Subsystem  TreatAsAtomicUnit=on
  If1 : If  IfExpression=(u1 == 0)
  NormalOp_LED : Subsystem  TreatAsAtomicUnit=on
  wires:
  If1/2 -> Fault_LED/Action
  Data Store Read1/1 -> If1/1
  If1/1 -> NormalOp_LED/Action

== system s32k344_mcb_open_loop_s32ct/Microcontroller/HW INT ==
  CodeGeneration : Subsystem  VariantControl=(codegen)
  Simulation : Subsystem  VariantControl=(sim)
  INT : Outport  OutputFunctionCall=on

== system s32k344_mcb_open_loop_s32ct/Microcontroller/Initialize Function ==
  Enable LCU : Subsystem  Priority=3
  Event Listener : EventListener  DisableCoverage=on  EventName=reset
  TPP Config : mbd_s32k3_utility_library/TPP Blocks/TPP Config  inst=0  desat_mode=off  full_mode=on  locks_mode=on  dead_time=500  overtemp_int=on  desat_int=on  vls_undervol_int=on  overcurr_int=on  phase_err_int=on  frame_err_int=on  write_err_int=on  rst_ev_int=on  en1_chn=GD_EN  en2_chn=GD_EN  rst_chn=GD_RST  cs_chn=GD_CS  spi_chn=GD3000_SPI  spi_seq=GD3000_SpiReadSequence
      settings: SourceProductName=Utility Blocks

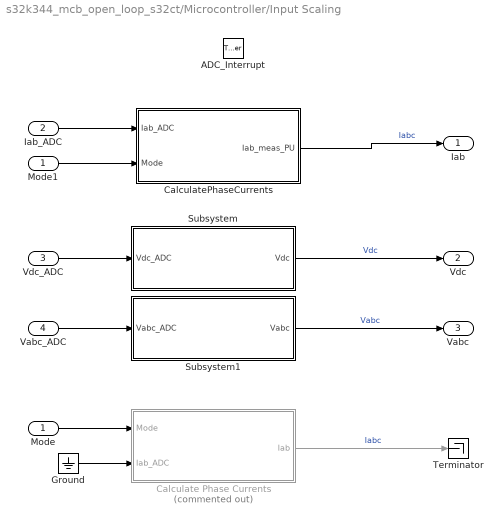
== system s32k344_mcb_open_loop_s32ct/Microcontroller/Input Scaling ==
  Mode : Inport
  Iab_ADC : Inport  Port=2
  Vdc_ADC : Inport  Port=3
  Vabc_ADC : Inport  Port=4
  ADC_Interrupt : TriggerPort  TriggerType=function-call  VariantControl=(inherit)
  Calculate Phase Currents : Subsystem  Commented=on  Variant=on
  CalculatePhaseCurrents : Subsystem  Priority=0
  Ground : Ground
  Mode1 : InportShadow
  Subsystem : Subsystem
  Subsystem1 : Subsystem
  Terminator : Terminator
  Iab : Outport
  Vdc : Outport  Port=2
  Vabc : Outport  Port=3
  wires:
  Iab_ADC/1 -> CalculatePhaseCurrents/1(Iab_ADC)
  Vdc_ADC/1 -> Subsystem/1(Vdc_ADC)
  Subsystem/1(Vdc) -> Vdc/1  "Vdc"
  CalculatePhaseCurrents/1(Iab_meas_PU) -> Iab/1  "Iabc"
  Vabc_ADC/1 -> Subsystem1/1(Vabc_ADC)
  Subsystem1/1(Vabc) -> Vabc/1  "Vabc"
  Mode/1 -> Calculate Phase Currents/1(Mode)
  Calculate Phase Currents/1(Iab) -> Terminator/1  "Iabc"
  Ground/1 -> Calculate Phase Currents/2(Iab_ADC)
  Mode1/1 -> CalculatePhaseCurrents/2(Mode)

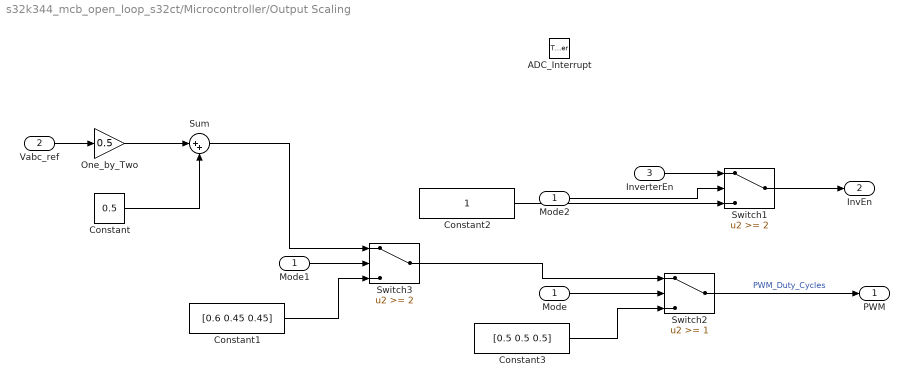
== system s32k344_mcb_open_loop_s32ct/Microcontroller/Output Scaling ==
  Mode : Inport
  Vabc_ref : Inport  Port=2
  InverterEn : Inport  Port=3
  ADC_Interrupt : TriggerPort  TriggerType=function-call  VariantControl=(inherit)
  Constant : Constant  Value=0.5  OutDataTypeStr=dataType  SampleTime=-1
  Constant1 : Constant  Value=[0.6 0.45 0.45]  OutDataTypeStr=dataType  SampleTime=-1
  Constant2 : Constant  OutDataTypeStr=dataType  SampleTime=-1
  Constant3 : Constant  Value=[0.5 0.5 0.5]  OutDataTypeStr=dataType  SampleTime=-1
  Mode1 : InportShadow
  Mode2 : InportShadow
  One_by_Two : Gain  Gain=0.5  RndMeth=Simplest  OutDataTypeStr=Inherit: Same as input
  Sum : Sum  Inputs=|++
  Switch1 : Switch  Threshold=2  SaturateOnIntegerOverflow=off  InputSameDT=off
  Switch2 : Switch  Threshold=1  SaturateOnIntegerOverflow=off  InputSameDT=off
  Switch3 : Switch  Threshold=2  SaturateOnIntegerOverflow=off  InputSameDT=off
  PWM : Outport
  InvEn : Outport  Port=2
  wires:
  Switch2/1 -> PWM/1  "PWM_Duty_Cycles"
  Constant/1 -> Sum/2
  One_by_Two/1 -> Sum/1
  InverterEn/1 -> Switch1/1
  Vabc_ref/1 -> One_by_Two/1
  Switch1/1 -> InvEn/1
  Constant2/1 -> Switch1/3
  Mode/1 -> Switch2/2
  Constant3/1 -> Switch2/3
  Switch3/1 -> Switch2/1
  Mode1/1 -> Switch3/2
  Constant1/1 -> Switch3/3
  Sum/1 -> Switch3/1
  Mode2/1 -> Switch1/2

== system s32k344_mcb_open_loop_s32ct/Microcontroller/SCIAbstraction ==
  SCI_Data : Inport
  Mode : Inport  Port=2
  SCI In Abstraction : Subsystem  ReferencedSubsystem=SCIInAbstractionOpenLoop
  ConfigAndCommand : Outport
  DebugSel : Outport  Port=2
  wires:
  SCI_Data/1 -> SCI In Abstraction/1
  Mode/1 -> SCI In Abstraction/2
  SCI In Abstraction/1 -> ConfigAndCommand/1
  SCI In Abstraction/2 -> DebugSel/1

== system s32k344_mcb_open_loop_s32ct/Microcontroller/SerialReceive ==
  Variant Subsystem : Subsystem  Variant=on  VariantControlMode=sim codegen switching
  Data : Outport
  wires:
  Variant Subsystem/1(Data) -> Data/1

== system s32k344_mcb_open_loop_s32ct/Microcontroller/SerialTransmit ==
  SerialData : Inport
  Constant : Constant  Value=uint8('S')  OutDataTypeStr=uint8
  Constant1 : Constant  Value=uint8('E')  OutDataTypeStr=uint8
  Terminator : Terminator
  Uart : mbd_s32k3_cdd_library/Uart  api_func=Uart_AsyncSend  channel=UartChannel_6  baudrate=UART_BAUDRATE_1200  transfer_type=UART_SEND  timeout=1e4  text=<binary blob, 3404 chars, not shown>
      settings: SourceProductName=CDD Blocks
  Vector Concatenate : Concatenate  NumInputs=3
  wires:
  Uart/1 -> Terminator/1
  Constant/1 -> Vector Concatenate/1
  Constant1/1 -> Vector Concatenate/3
  Vector Concatenate/1 -> Uart/1
  SerialData/1 -> Vector Concatenate/2

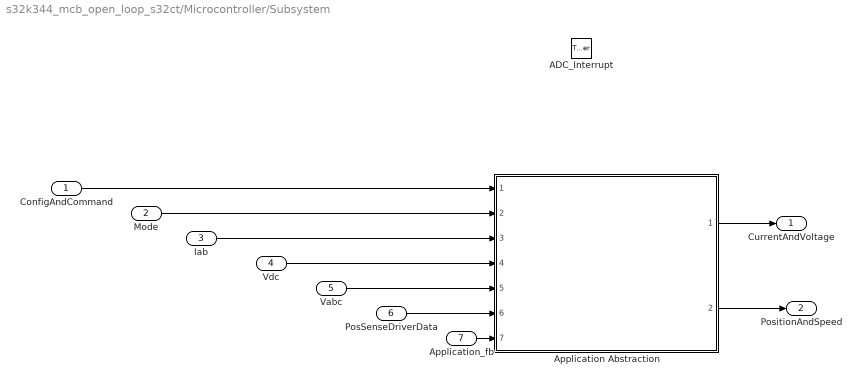
== system s32k344_mcb_open_loop_s32ct/Microcontroller/Subsystem ==
  ConfigAndCommand : Inport
  Mode : Inport  Port=2
  Iab : Inport  Port=3
  Vdc : Inport  Port=4
  Vabc : Inport  Port=5
  PosSenseDriverData : Inport  Port=6
  Application_fb : Inport  Port=7
  ADC_Interrupt : TriggerPort  TriggerType=function-call  VariantControl=(inherit)
  Application Abstraction : Subsystem  ReferencedSubsystem=ApplicationAbstractionOpenLoop
  CurrentAndVoltage : Outport
  PositionAndSpeed : Outport  Port=2
  wires:
  Application Abstraction/1 -> CurrentAndVoltage/1
  PosSenseDriverData/1 -> Application Abstraction/6
  ConfigAndCommand/1 -> Application Abstraction/1
  Application Abstraction/2 -> PositionAndSpeed/1
  Mode/1 -> Application Abstraction/2
  Application_fb/1 -> Application Abstraction/7
  Vabc/1 -> Application Abstraction/5
  Vdc/1 -> Application Abstraction/4
  Iab/1 -> Application Abstraction/3

== system s32k344_mcb_open_loop_s32ct/Microcontroller/Subsystem1 ==
  IabADCIn : Inport
  eQEPIn : Inport  Port=2
  ADC_Interrupt : TriggerPort  TriggerType=function-call  VariantControl=(inherit)
  Input HW Drivers : Subsystem  Variant=on  VariantControlMode=sim codegen switching
  IabADC : Outport
  VdcADC : Outport  Port=2
  Vabc_ADC : Outport  Port=3
  eQEP : Outport  Port=4
  wires:
  Input HW Drivers/1(IabADC) -> IabADC/1
  Input HW Drivers/3(Vabc_ADC) -> Vabc_ADC/1
  Input HW Drivers/4(eQEP) -> eQEP/1
  Input HW Drivers/2(VdcADC) -> VdcADC/1
  eQEPIn/1 -> Input HW Drivers/2(eQEPIn)
  IabADCIn/1 -> Input HW Drivers/1(IabADCIn)

== system s32k344_mcb_open_loop_s32ct/Microcontroller/Subsystem2 ==
  PWM In : Inport
  InvEn : Inport  Port=2
  ADC_Interrupt : TriggerPort  TriggerType=function-call  VariantControl=(inherit)
  Output PWM Drivers : Subsystem  Variant=on  VariantControlMode=sim codegen switching
  PWM : Outport
  wires:
  Output PWM Drivers/1(PWM) -> PWM/1
  InvEn/1 -> Output PWM Drivers/2(InvEn)
  PWM In/1 -> Output PWM Drivers/1(PWM In)

== system s32k344_mcb_open_loop_s32ct/Inverter and Motor/Inverter and Motor/Codegen ==
  Duty_Cycles : Inport
  Data Type Conversion : DataTypeConversion  OutDataTypeStr=uint16  RndMeth=Simplest  SaturateOnIntegerOverflow=off
  Data Type Conversion1 : DataTypeConversion  OutDataTypeStr=uint16  RndMeth=Simplest  SaturateOnIntegerOverflow=off
  Ground : Ground
  Ground1 : Ground
  Terminator : Terminator
  PhaseCurr_fb : Outport
  Position_fb : Outport  Port=2
  wires:
  Duty_Cycles/1 -> Terminator/1
  Ground/1 -> Data Type Conversion/1
  Ground1/1 -> Data Type Conversion1/1
  Data Type Conversion/1 -> PhaseCurr_fb/1
  Data Type Conversion1/1 -> Position_fb/1

== system s32k344_mcb_open_loop_s32ct/Inverter and Motor/Inverter and Motor/Sim ==
  Duty_Cycles : Inport
  Motor : Subsystem  ReferencedSubsystem=MotorPMSMOpenLoop
  Rate Transition3 : RateTransition  Deterministic=off  OutPortSampleTime=Ts_inverter
  Subsystem : Subsystem
  PhaseCurr_fb : Outport
  Position_fb : Outport  Port=2
  wires:
  Duty_Cycles/1 -> Rate Transition3/1
  Motor/1 -> Subsystem/1(Iabc)
  Motor/2 -> Subsystem/2(ThetaMech)
  Subsystem/2(eQEP) -> Position_fb/1
  Subsystem/1(IabADC) -> PhaseCurr_fb/1
  Rate Transition3/1 -> Motor/1

== system s32k344_mcb_open_loop_s32ct/Microcontroller/BoardLEDs/Fault_LED ==
  Action Port : ActionPort  ActionPortLabel=else
  Constant : Constant  OutDataTypeStr=uint8
  Constant1 : Constant  Value=0  OutDataTypeStr=uint8
  Constant2 : Constant  Value=0  OutDataTypeStr=uint8
  Dio : mbd_s32k3_io_library/Dio  api_func=Dio_WriteChannel  channel=RGBLED0_RED  channel_group=No channel groups configured  port=PTA_H  gpioSim=on  text=<binary blob, 4674 chars, not shown>
      settings: SourceProductName=IO Blocks
  Dio1 : mbd_s32k3_io_library/Dio  api_func=Dio_WriteChannel  channel=RGBLED0_GREEN  channel_group=No channel groups configured  port=PTA_H  gpioSim=on  text=<binary blob, 4674 chars, not shown>
      settings: SourceProductName=IO Blocks
  Dio2 : mbd_s32k3_io_library/Dio  api_func=Dio_WriteChannel  channel=RGBLED0_BLUE  channel_group=No channel groups configured  port=PTA_H  gpioSim=on  text=<binary blob, 4674 chars, not shown>
      settings: SourceProductName=IO Blocks
  wires:
  Constant/1 -> Dio/1
  Constant1/1 -> Dio1/1
  Constant2/1 -> Dio2/1

== system s32k344_mcb_open_loop_s32ct/Microcontroller/BoardLEDs/NormalOp_LED ==
  Action Port : ActionPort  ActionPortLabel=if((u1 == 0))
  Data Store Read : DataStoreRead  DataStoreName=Enable  IndexOptions=Index vector (dialog)  Indices=1  OutputSizes=1
  If : If  IfExpression=u1 == 1
  If Action Subsystem : Subsystem  TreatAsAtomicUnit=on
  If Action Subsystem1 : Subsystem  TreatAsAtomicUnit=on
  wires:
  Data Store Read/1 -> If/1
  If/1 -> If Action Subsystem/Action
  If/2 -> If Action Subsystem1/Action

== system s32k344_mcb_open_loop_s32ct/Microcontroller/HW INT/CodeGeneration ==
  ADC_INT : Subsystem  TreatAsAtomicUnit=on
  INT : Outport
  wires:
  ADC_INT/1(FcnCall) -> INT/1

== system s32k344_mcb_open_loop_s32ct/Microcontroller/HW INT/Simulation ==
  ADC_INT : simulink/Ports & Subsystems/Function-Call Generator  sample_time=Ts  numberOfIterations=1  DisallowWideOutput=off
  INT : Outport  OutputFunctionCall=on
  wires:
  ADC_INT/1 -> INT/1

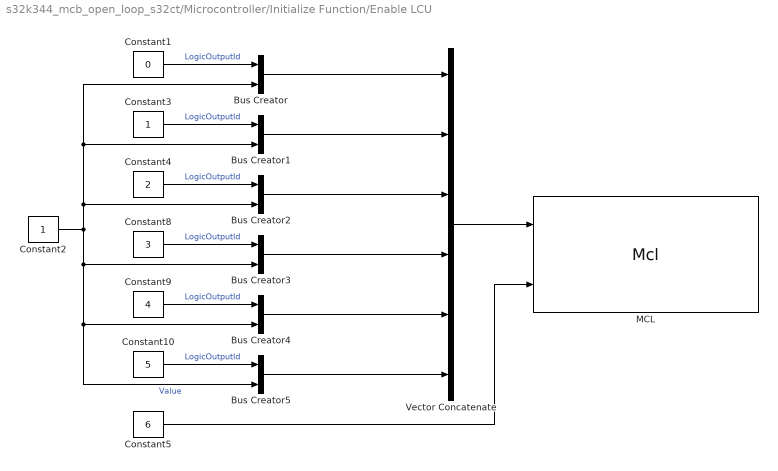
== system s32k344_mcb_open_loop_s32ct/Microcontroller/Initialize Function/Enable LCU ==
  Bus Creator{,1..5} (6 alike) : BusCreator  Inputs=LogicOutputId,Value  OutDataTypeStr=Bus: Mcl_LcuSyncOutputValueType  NonVirtualBus=on
  Constant1 : Constant  Value=0  OutDataTypeStr=uint8
  Constant10 : Constant  Value=5  OutDataTypeStr=uint8
  Constant2 : Constant  OutDataTypeStr=uint16
  Constant3 : Constant  OutDataTypeStr=uint8
  Constant4 : Constant  Value=2  OutDataTypeStr=uint8
  Constant5 : Constant  Value=6  OutDataTypeStr=uint8
  Constant8 : Constant  Value=3  OutDataTypeStr=uint8
  Constant9 : Constant  Value=4  OutDataTypeStr=uint8
  MCL : mbd_s32k3_cdd_library/Mcl  Priority=2  api_func=Mcl_SetLcuSyncOutputEnable  logicInput=LCU_LOGIC_INPUT_0  logicOutput=LCU_LOGIC_OUTPUT_0  logicInstance=LCU_LOGIC_INSTANCE_0  emiosInstance=EMIOS_0  ftmInstance=FTM0  logicChannel=EMIOS_0_EmiosMclMasterBus_0  prescalerType=MCL_EMIOS_PRESCALER  dmaLogicInstance=No DMA logic instances configured  dmaLogicChannel=DMA_LOGIC_CH_0  dmaInstanceCommandType=MCL_DMA_INST_STOP  dmaChannelCommandType=MCL_DMA_CH_START_REQUEST  dmaScatterGatherElement=No DMA Scatter Gather elements configured  dmaChannelInfo=MCL_DMA_CH_GET_SOURCE_ADDRESS  text=<binary blob, 55810 chars, not shown>
      settings: SourceProductName=CDD Blocks
  Vector Concatenate : Concatenate  NumInputs=6
  wires:
  Constant4/1 -> Bus Creator2/1  "LogicOutputId"
  Constant2/1 -> Bus Creator/2, Bus Creator1/2, Bus Creator2/2, Bus Creator5/2, Bus Creator4/2, Bus Creator3/2  "Value"
  Constant1/1 -> Bus Creator/1  "LogicOutputId"
  Bus Creator4/1 -> Vector Concatenate/5
  Constant9/1 -> Bus Creator4/1  "LogicOutputId"
  Bus Creator/1 -> Vector Concatenate/1
  Constant5/1 -> MCL/2
  Constant8/1 -> Bus Creator3/1  "LogicOutputId"
  Bus Creator2/1 -> Vector Concatenate/3
  Constant10/1 -> Bus Creator5/1  "LogicOutputId"
  Bus Creator5/1 -> Vector Concatenate/6
  Vector Concatenate/1 -> MCL/1
  Constant3/1 -> Bus Creator1/1  "LogicOutputId"
  Bus Creator1/1 -> Vector Concatenate/2
  Bus Creator3/1 -> Vector Concatenate/4

== system s32k344_mcb_open_loop_s32ct/Microcontroller/Input Scaling/Calculate Phase Currents ==
  Mode : Inport
  Iab_ADC : Inport  Port=2
  Automatic offset calibration : Subsystem  VariantControl=inverter.ADCOffsetCalibEnable == 1
  Offser via parameter : Subsystem  VariantControl=inverter.ADCOffsetCalibEnable == 0
  Iab : Outport

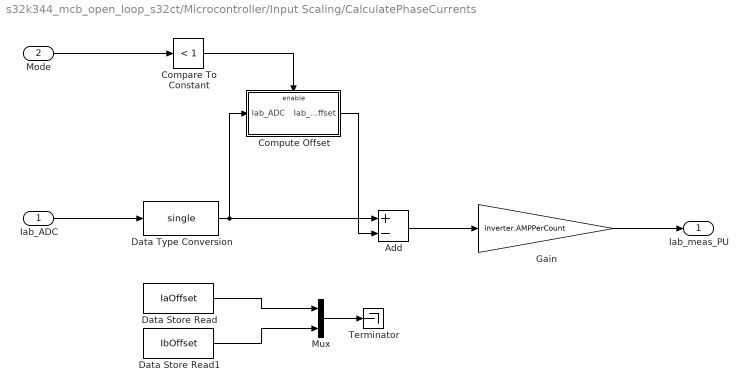
== system s32k344_mcb_open_loop_s32ct/Microcontroller/Input Scaling/CalculatePhaseCurrents ==
  Iab_ADC : Inport
  Mode : Inport  Port=2
  Add : Sum  Inputs=+-
  Compare To Constant : simulink/Logic and Bit Operations/Compare To Constant  relop=<  const=1  OutDataTypeStr=boolean
  Compute Offset : Subsystem
  Data Store Read : DataStoreRead  DataStoreName=IaOffset  IndexOptions=Index vector (dialog)  Indices=1  OutputSizes=1
  Data Store Read1 : DataStoreRead  DataStoreName=IbOffset  IndexOptions=Index vector (dialog)  Indices=1  OutputSizes=1
  Data Type Conversion : DataTypeConversion  OutDataTypeStr=single  SaturateOnIntegerOverflow=off  RndMeth=Floor
  Gain : Gain  Gain=inverter.AMPPerCount  RndMeth=Simplest  OutDataTypeStr=Inherit: Same as input
  Mux : Mux  Inputs=2
  Terminator : Terminator
  Iab_meas_PU : Outport
  wires:
  Iab_ADC/1 -> Data Type Conversion/1
  Data Store Read/1 -> Mux/1
  Data Store Read1/1 -> Mux/2
  Add/1 -> Gain/1
  Gain/1 -> Iab_meas_PU/1
  Compare To Constant/1 -> Compute Offset/Enable
  Mode/1 -> Compare To Constant/1
  Data Type Conversion/1 -> Compute Offset/1(Iab_ADC), Add/1
  Compute Offset/1(Iab_Offset) -> Add/2
  Mux/1 -> Terminator/1

== system s32k344_mcb_open_loop_s32ct/Microcontroller/Input Scaling/Subsystem ==
  Vdc_ADC : Inport
  Gain : Gain  Gain=inverter.VoltPerCount  OutDataTypeStr=dataType  RndMeth=Simplest
  Vdc : Outport
  wires:
  Gain/1 -> Vdc/1
  Vdc_ADC/1 -> Gain/1

== system s32k344_mcb_open_loop_s32ct/Microcontroller/Input Scaling/Subsystem1 ==
  Vabc_ADC : Inport
  Gain : Gain  Gain=inverter.VoltPerCount  OutDataTypeStr=dataType  RndMeth=Simplest
  Vabc : Outport
  wires:
  Gain/1 -> Vabc/1
  Vabc_ADC/1 -> Gain/1

== system s32k344_mcb_open_loop_s32ct/Microcontroller/SerialReceive/Variant Subsystem ==
  CodeGeneration : Subsystem  VariantControl=(codegen)
  Simulation : Subsystem  VariantControl=(sim)
  Data : Outport

== system s32k344_mcb_open_loop_s32ct/Microcontroller/Subsystem1/Input HW Drivers ==
  IabADCIn : Inport
  eQEPIn : Inport  Port=2
  Codegen : Subsystem  VariantControl=(codegen)
  Sim : Subsystem  VariantControl=(sim)
  IabADC : Outport
  VdcADC : Outport  Port=2
  Vabc_ADC : Outport  Port=3
  eQEP : Outport  Port=4

== system s32k344_mcb_open_loop_s32ct/Microcontroller/Subsystem2/Output PWM Drivers ==
  PWM In : Inport
  InvEn : Inport  Port=2
  Codegen : Subsystem  VariantControl=(codegen)
  Sim : Subsystem  VariantControl=(sim)
  PWM : Outport

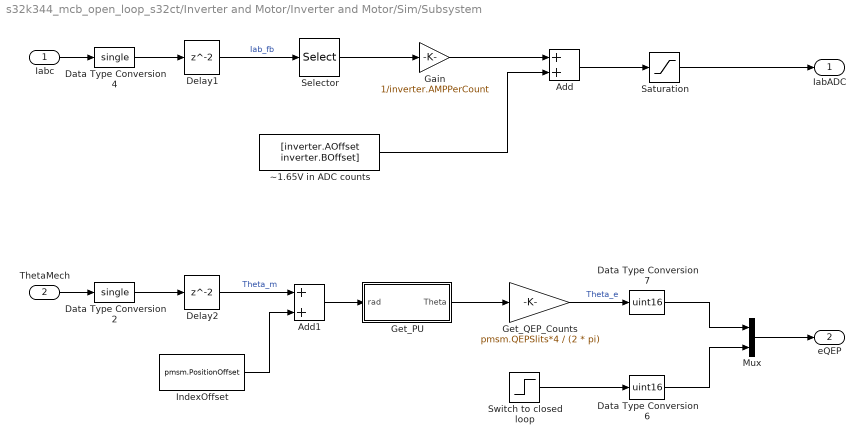
== system s32k344_mcb_open_loop_s32ct/Inverter and Motor/Inverter and Motor/Sim/Subsystem ==
  Iabc : Inport
  ThetaMech : Inport  Port=2
  Add : Sum  RndMeth=Simplest  OutDataTypeStr=Inherit: Same as first input
  Add1 : Sum  RndMeth=Simplest
  Data Type Conversion2 : DataTypeConversion  OutDataTypeStr=single  RndMeth=Simplest  SaturateOnIntegerOverflow=off
  Data Type Conversion4 : DataTypeConversion  OutDataTypeStr=single  RndMeth=Simplest  SaturateOnIntegerOverflow=off
  Data Type Conversion6 : DataTypeConversion  OutDataTypeStr=uint16  RndMeth=Simplest  SaturateOnIntegerOverflow=off
  Data Type Conversion7 : DataTypeConversion  OutDataTypeStr=uint16  RndMeth=Simplest  SaturateOnIntegerOverflow=off
  Delay1 : Delay
  Delay2 : Delay
  Gain : Gain  Gain=1/inverter.AMPPerCount  OutDataTypeStr=int16
  "Get_PU " : Subsystem
  Get_QEP_Counts : Gain  Gain=pmsm.QEPSlits*4 / (2 * pi)  OutDataTypeStr=uint16  RndMeth=Simplest
  IndexOffset : Constant  Value=pmsm.PositionOffset  OutDataTypeStr=single  SampleTime=-1
  Mux : Mux  Inputs=2
  Saturation : Saturate  UpperLimit=inverter.MaxADCCnt  LowerLimit=0  OutDataTypeStr=uint16  RndMeth=Simplest
  Selector : Selector  InputPortWidth=3  IndexOptions=Index vector (dialog)  Indices=[1 2]  OutputSizes=1
  "Switch to closed loop " : Step  Time=0.1  SampleTime=Ts_motor
  ~1.65V in ADC counts : Constant  Value=[inverter.AOffset inverter.BOffset]  OutDataTypeStr=uint16  SampleTime=-1
  IabADC : Outport
  eQEP : Outport  Port=2
  wires:
  "Switch to closed loop "/1 -> Data Type Conversion6/1
  Iabc/1 -> Data Type Conversion4/1
  Get_QEP_Counts/1 -> Data Type Conversion7/1  "Theta_e"
  Mux/1 -> eQEP/1
  Data Type Conversion6/1 -> Mux/2
  Delay1/1 -> Selector/1  "Iab_fb"
  "Get_PU "/1(Theta) -> Get_QEP_Counts/1
  IndexOffset/1 -> Add1/2
  Data Type Conversion7/1 -> Mux/1
  Data Type Conversion2/1 -> Delay2/1
  Data Type Conversion4/1 -> Delay1/1
  ThetaMech/1 -> Data Type Conversion2/1
  Saturation/1 -> IabADC/1
  Selector/1 -> Gain/1
  Gain/1 -> Add/1
  ~1.65V in ADC counts/1 -> Add/2
  Add/1 -> Saturation/1
  Delay2/1 -> Add1/1  "Theta_m"
  Add1/1 -> "Get_PU "/1(rad)

== system s32k344_mcb_open_loop_s32ct/Microcontroller/BoardLEDs/NormalOp_LED/If Action Subsystem ==
  Action Port : ActionPort  ActionPortLabel=if(u1 == 1)
  Constant : Constant  OutDataTypeStr=uint8
  Constant1 : Constant  Value=0  OutDataTypeStr=uint8
  Constant2 : Constant  Value=0  OutDataTypeStr=uint8
  Dio : mbd_s32k3_io_library/Dio  api_func=Dio_WriteChannel  channel=RGBLED0_GREEN  channel_group=No channel groups configured  port=PTA_H  gpioSim=on  text=<binary blob, 4674 chars, not shown>
      settings: SourceProductName=IO Blocks
  Dio1 : mbd_s32k3_io_library/Dio  api_func=Dio_WriteChannel  channel=RGBLED0_BLUE  channel_group=No channel groups configured  port=PTA_H  gpioSim=on  text=<binary blob, 4674 chars, not shown>
      settings: SourceProductName=IO Blocks
  Dio2 : mbd_s32k3_io_library/Dio  api_func=Dio_WriteChannel  channel=RGBLED0_RED  channel_group=No channel groups configured  port=PTA_H  gpioSim=on  text=<binary blob, 4674 chars, not shown>
      settings: SourceProductName=IO Blocks
  wires:
  Constant1/1 -> Dio1/1
  Constant/1 -> Dio/1
  Constant2/1 -> Dio2/1

== system s32k344_mcb_open_loop_s32ct/Microcontroller/BoardLEDs/NormalOp_LED/If Action Subsystem1 ==
  Action Port : ActionPort  ActionPortLabel=else
  Constant : Constant  Value=0  OutDataTypeStr=uint8
  Constant1 : Constant  Value=0  OutDataTypeStr=uint8
  Constant2 : Constant  OutDataTypeStr=uint8
  Dio : mbd_s32k3_io_library/Dio  api_func=Dio_WriteChannel  channel=RGBLED0_GREEN  channel_group=No channel groups configured  port=PTA_H  gpioSim=on  text=<binary blob, 4674 chars, not shown>
      settings: SourceProductName=IO Blocks
  Dio1 : mbd_s32k3_io_library/Dio  api_func=Dio_WriteChannel  channel=RGBLED0_RED  channel_group=No channel groups configured  port=PTA_H  gpioSim=on  text=<binary blob, 4674 chars, not shown>
      settings: SourceProductName=IO Blocks
  Dio2 : mbd_s32k3_io_library/Dio  api_func=Dio_WriteChannel  channel=RGBLED0_BLUE  channel_group=No channel groups configured  port=PTA_H  gpioSim=on  text=<binary blob, 4674 chars, not shown>
      settings: SourceProductName=IO Blocks
  wires:
  Constant1/1 -> Dio1/1
  Constant/1 -> Dio/1
  Constant2/1 -> Dio2/1
